simulink model "holtsav_figyelmen_kivul_hagyasanak_hatasa"  (Simulink 8.7)
settings: Solver=VariableStepAuto  StartTime=0.0  StopTime=T_sim  RelTol=1e-3
values from neighbouring files (symbols this model uses):
  K_C = 1/P1d.Numerator(2)*(1-exp(-Ts/T_cl))    [Sebessegszabalyozas_sim.m]
  P1d = c2d(sys,Ts,'zoh')    [Sebessegszabalyozas_sim.m]
  Ts = 0.1    [Sebessegszabalyozas_sim.m]
  u_sat = y_sat/K    [Sebessegszabalyozas_sim.m]
  u_stat = [0;100;200;250;300;350;400;450;500;550;600;700;750]    [Untitled.m]    (also in ident.mat = [0 100 200 300 400 500 600 700])
  y_stat = y_stat*K    [Sebessegszabalyozas_sim.m]    (also in Untitled.m = [0;  0;  0;  0; 42; 67; 80; 95;110;120;130;160;170]; ident.mat = [0 0 0 32 100 160 216 260])
  z_d = -P1d.Denominator(2)    [Sebessegszabalyozas_sim.m]
settings Model: Creator=Mester Ádám  LastModifiedBy=Mester Ádám
settings DataIOCC: LimitDataPoints=off  SaveFormat=Dataset
settings DebuggingCC: UnderspecifiedInitializationDetection=Simplified  MergeDetectMultiDrivingBlocksExec=error
settings HardwareCC: ProdBitPerPointer=64  ProdLargestAtomicFloat=Float  ProdIntDivRoundTo=Zero  ProdEndianess=LittleEndian  ProdWordSize=64  ProdHWDeviceType=Intel->x86-64 (Windows64)
settings ModelReferenceCC: PropagateSignalLabelsOutOfModel=on
settings ConfigComp: CovModelRefEnable=off

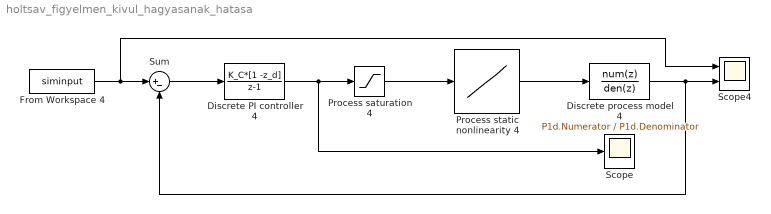
== system holtsav_figyelmen_kivul_hagyasanak_hatasa ==
  Discrete PI controller 4 : DiscreteTransferFcn  Numerator=K_C*[1 -z_d]  Denominator=[1 -1]  SampleTime=Ts
  Discrete process model 4 : DiscreteTransferFcn  Numerator=P1d.Numerator  Denominator=P1d.Denominator  SampleTime=Ts
  From Workspace 4 : FromWorkspace  VariableName=siminput  SampleTime=Ts
  Process saturation 4 : Saturate  UpperLimit=u_sat  LowerLimit=0
  Process static nonlinearity 4 : Lookup_n-D  NumberOfTableDimensions=1  BreakpointsForDimension1=u_stat  Table=y_stat  InternalRulePriority=Speed  RndMeth=Simplest  InputSameDT=on
  Scope : Scope
  Scope4 : Scope  NumInputPorts=2
  Sum : Sum  Inputs=|+-
  wires:
  Discrete process model 4/1 -> Sum/2, Scope4/2
  From Workspace 4/1 -> Sum/1, Scope4/1
  Sum/1 -> Discrete PI controller 4/1
  Discrete PI controller 4/1 -> Process saturation 4/1, Scope/1
  Process static nonlinearity 4/1 -> Discrete process model 4/1
  Process saturation 4/1 -> Process static nonlinearity 4/1
